simulink model "METI_Thermal_ver01_Jmaab_2018b"  (R2018b)
settings: Solver=ode8  StartTime=0  StopTime=end_time  FixedStep=sampling_time  RelTol=1e-3
PreLoadFcn:
  | %init_setting;
values from neighbouring files (symbols this model uses):
  degC2K = 273.15    [METI_TRAMI_Thermal_ver01_Jmaab_PreLoad.m]    (also in init_setting_METI.m)
  K2degC = -273.15    [METI_TRAMI_Thermal_ver01_Jmaab_PreLoad.m]    (also in init_setting_METI.m)
  sampling_time = 0.0025    [METI_TRAMI_Thermal_ver01_Jmaab_PreLoad.m]
undefined symbols (not defined in the file or in its folder): ACC_D_Gain, ACC_I_Gain, ACC_P_Gain, ALT_CNT_ALT_OFF_RPM_HYS_rpm, ALT_CNT_ALT_ON_RPM_HYS_rpm, ALT_CNT_Alter_V_BASE_V, ALT_CNT_Alter_V_Kaisei_V, ALT_CNT_flag_disable_kaisei, ALT_CNT_V_Battely_Kudo_V, ALT_PNT_ALT_GDCurrent_A, ALT_PNT_ALT_GDVolt_V, ALT_PNT_Alter_limit_Current_V_table, ALT_PNT_Alter_limit_Current_V_table_x_rpm, ALT_PNT_Alter_trq_Nm_map, ALT_PNT_Alter_trq_Nm_map_x_rpm, ALT_PNT_Alter_trq_Nm_map_y_Current_A, ALT_PNT_Alter_trq_Nm_map_z_Volt_tgt_V, ALT_PNT_eta_pulley_alt, ALT_PNT_Gain_Alt_v_del, ALT_PNT_ratio_pulley_alt, ALT_PNT_Tau_Alternator_V_tgt_s, ALT_PNT_trq_alter_output_LL_Nm, BK_PNT_Pow_UL, BK_PNT_Tau_brake, Brk_LL, Brk_PGain, Brk_UL, BT_PNT_Lo_Capa_lo_batt_F, BT_PNT_Lo_ocv_SOC_lo_batt_OCV_V_table, BT_PNT_Lo_ocv_SOC_lo_batt_OCV_V_table_x_SOC, BT_PNT_Lo_R_lo_batt_ohm, BT_PNT_Lo_SOC_MAX_lo_batt, BT_PNT_Lo_SOC_MIN_lo_batt, BT_PNT_Lo_SOC_START_lo_batt, BT_PNT_Lo_V_start_ocv, DF_PNT_DF_gear, DF_PNT_DFBlock2DFAir_Heat_Resi_KpW, DF_PNT_DFBlock_Heat_Capa_JpK, DF_PNT_DFBlock_Temp_ini_degC, DF_PNT_DFOil2DFBlock_Heat_Resi_KpW, DF_PNT_DFOil_Heat_Capa_JpK, DF_PNT_DFOil_Temp_ini_degC, DF_PNT_Driveshaft_damper, DF_PNT_Driveshaft_delta_radps_LL, DF_PNT_Driveshaft_delta_radps_UL, DF_PNT_Driveshaft_spring, DF_PNT_eta_DF, DF_PNT_Outtemp_degC, DF_PNT_TMBlock2DFBlock_Heat_Resi_KpW, Driver_Brake_Const1, Driver_Brake_Const3, Driver_Brake_Switch_Const2, Driver_Brk_sh, drivmode_ACC, drivmode_CONST, drivmode_GensokuKaisei, drivmode_GensokuRikko, drivmode_STOP, EL_PNT_R_bodyelec_lo_ohm, ENG_CNT_acc_idlestop ... (+137)
libraries: METI_Lib_vehicle_model x31, simulink x7, AZAPA_Lib_vehicle_model x1
(part 4 of 4)

== system METI_Thermal_ver01_Jmaab_2018b/Vehicle/CNT/ENG_CNT/ENG_Cntrl/Caliculate_Idle_Speed/Subsystem1 ==
  note: アイドル回転数時のFB
  omg_tgt_idle : Inport
  n_eng_rpm : Inport  Port=2
  per_throttle_base : Inport  Port=3
  flag_Lockup : Inport  Port=4
  flag_IdleStop : Inport  Port=5
  Logical Operator : Logic  Operator=OR  AllPortsSameDT=off  OutDataTypeStr=boolean
  Logical Operator1 : Logic  Operator=NOT  AllPortsSameDT=off  OutDataTypeStr=boolean
  Logical Operator2 : Logic  Inputs=3  AllPortsSameDT=off  OutDataTypeStr=boolean
  Logical Operator3 : Logic  Operator=NOT  AllPortsSameDT=off  OutDataTypeStr=boolean
  Logical Operator4 : Logic  Operator=NOT  AllPortsSameDT=off  OutDataTypeStr=boolean
  Logical Operator5 : Logic  AllPortsSameDT=off  OutDataTypeStr=boolean
  Relational Operator : RelationalOperator  Operator=<  OutDataTypeStr=boolean  RndMeth=Nearest
  Relational Operator2 : RelationalOperator  Operator=>  OutDataTypeStr=boolean  RndMeth=Nearest
  per_throttle_isc_fb : Constant  Value=ENG_CNT_per_throttle_isc_fb
  flag_idle_fb : Outport
  wires:
  per_throttle_base/1 -> Relational Operator/1
  per_throttle_isc_fb/1 -> Relational Operator/2
  Relational Operator2/1 -> Logical Operator2/1
  Relational Operator/1 -> Logical Operator1/1, Logical Operator5/1
  Logical Operator1/1 -> Logical Operator2/2
  Logical Operator5/1 -> Logical Operator/2
  flag_Lockup/1 -> Logical Operator3/1
  Logical Operator3/1 -> Logical Operator2/3
  Logical Operator2/1 -> Logical Operator/1
  omg_tgt_idle/1 -> Relational Operator2/1
  n_eng_rpm/1 -> Relational Operator2/2
  flag_IdleStop/1 -> Logical Operator4/1
  Logical Operator4/1 -> Logical Operator5/2
  Logical Operator/1 -> flag_idle_fb/1

== system METI_Thermal_ver01_Jmaab_2018b/Vehicle/PTTH/DTTH_PNT/DFTH_PNT/DFBlock_Heat_Capacity/degC->K ==
  degC : Inport
  Constant2 : Constant  Value=degC2K
  Sum : Sum  Inputs=++|
  K : Outport
  wires:
  degC/1 -> Sum/2
  Constant2/1 -> Sum/1
  Sum/1 -> K/1

== system METI_Thermal_ver01_Jmaab_2018b/Vehicle/PTTH/DTTH_PNT/DFTH_PNT/DFOil_Heat_Capacity/degC->K ==
  degC : Inport
  Constant2 : Constant  Value=degC2K
  Sum : Sum  Inputs=++|
  K : Outport
  wires:
  degC/1 -> Sum/2
  Constant2/1 -> Sum/1
  Sum/1 -> K/1

== system METI_Thermal_ver01_Jmaab_2018b/Vehicle/PTTH/DTTH_PNT/TMTH_PNT/CVTF_Heat_Capacity/degC->K ==
  degC : Inport
  Constant2 : Constant  Value=degC2K
  Sum : Sum  Inputs=++|
  K : Outport
  wires:
  degC/1 -> Sum/2
  Constant2/1 -> Sum/1
  Sum/1 -> K/1

== system METI_Thermal_ver01_Jmaab_2018b/Vehicle/PTTH/DTTH_PNT/TMTH_PNT/TMBlock_Heat_Capacity/degC->K ==
  degC : Inport
  Constant2 : Constant  Value=degC2K
  Sum : Sum  Inputs=++|
  K : Outport
  wires:
  degC/1 -> Sum/2
  Constant2/1 -> Sum/1
  Sum/1 -> K/1

== system METI_Thermal_ver01_Jmaab_2018b/Vehicle/PTTH/ENGTH_PNT/Subsystem/Coolant_Heat_Capacity/degC->K ==
  degC : Inport
  Constant2 : Constant  Value=degC2K
  Sum : Sum  Inputs=++|
  K : Outport
  wires:
  degC/1 -> Sum/2
  Constant2/1 -> Sum/1
  Sum/1 -> K/1

== system METI_Thermal_ver01_Jmaab_2018b/Vehicle/PTTH/ENGTH_PNT/Subsystem/ENGBlock_Heat_Capacity/degC->K ==
  degC : Inport
  Constant2 : Constant  Value=degC2K
  Sum : Sum  Inputs=++|
  K : Outport
  wires:
  degC/1 -> Sum/2
  Constant2/1 -> Sum/1
  Sum/1 -> K/1

== system METI_Thermal_ver01_Jmaab_2018b/Vehicle/PTTH/ENGTH_PNT/Subsystem/ENGOil_Heat_Capacity/degC->K ==
  degC : Inport
  Constant2 : Constant  Value=degC2K
  Sum : Sum  Inputs=++|
  K : Outport
  wires:
  degC/1 -> Sum/2
  Constant2/1 -> Sum/1
  Sum/1 -> K/1

== system METI_Thermal_ver01_Jmaab_2018b/Vehicle/PTTH/ENGTH_PNT/Subsystem/ENGOil_Heat_Capacity1/degC->K ==
  degC : Inport
  Constant2 : Constant  Value=degC2K
  Sum : Sum  Inputs=++|
  K : Outport
  wires:
  degC/1 -> Sum/2
  Constant2/1 -> Sum/1
  Sum/1 -> K/1

== system METI_Thermal_ver01_Jmaab_2018b/Vehicle/PTTH/RDTH_PNT/Subsystem/ENGBlock2Coolant_Heat_Resistance/K->degC ==
  K : Inport
  Constant2 : Constant  Value=K2degC
  Sum : Sum  Inputs=++|
  degC : Outport
  wires:
  K/1 -> Sum/2
  Constant2/1 -> Sum/1
  Sum/1 -> degC/1

== system METI_Thermal_ver01_Jmaab_2018b/Vehicle/PTTH/RDTH_PNT/Subsystem/RDCoolant_Heat_Capacity/degC->K ==
  degC : Inport
  Constant2 : Constant  Value=degC2K
  Sum : Sum  Inputs=++|
  K : Outport
  wires:
  degC/1 -> Sum/2
  Constant2/1 -> Sum/1
  Sum/1 -> K/1

== system METI_Thermal_ver01_Jmaab_2018b/Vehicle/TM_PNT/TM_PNT/TC_PNT/T_C/Cal_C_Capacity ==
  note: 容量係数
      | 加速中は＋
      | 減速中は－
  note: capacity coefficient
  note: N・m/rpm2
  ratio_n : Inport
  flag_acc_del : Inport  Port=2
  Product2 : Product  RndMeth=Zero
  ×10＾-6 : Gain  Gain=TM_PNT_ConvUnit
  容量係数 Lookup Table1 : Lookup_n-D  NumberOfTableDimensions=1  BreakpointsForDimension1=TM_PNT_torque_capacity_Nmprpm2_table_x_speed_ratio  Table=TM_PNT_torque_capacity_Nmprpm2_table  RndMeth=Simplest  InputSameDT=on
  c_capacity : Outport
  wires:
  容量係数 Lookup Table1/1 -> ×10＾-6/1
  ×10＾-6/1 -> Product2/1
  ratio_n/1 -> 容量係数 Lookup Table1/1
  Product2/1 -> c_capacity/1
  flag_acc_del/1 -> Product2/2

== system METI_Thermal_ver01_Jmaab_2018b/Vehicle/TM_PNT/TM_PNT/TC_PNT/T_C/Cal_Ratio_n ==
  n_TM_PNT_rpm : Inport
  n_GR_rpm : Inport  Port=2
  Compare To Constant1 : simulink/Logic and Bit Operations/Compare To Constant  relop=<=  const=TM_PNT_n_TC_min_rpm  OutDataTypeStr=boolean
  Compare To Constant2 : simulink/Logic and Bit Operations/Compare To Constant  relop=<=  const=TM_PNT_n_TC_min_rpm  OutDataTypeStr=boolean
  Constant : Constant  Value=0
  Logical Operator1 : Logic  Operator=OR  AllPortsSameDT=off  OutDataTypeStr=boolean
  MinMax : MinMax  Inputs=2
  Saturation1 : Saturate  UpperLimit=TM_PNT_w_ROT_T_C_UL  LowerLimit=TM_PNT_w_ROT_T_C_LL
  Saturation2 : Saturate  UpperLimit=TM_PNT_w_ROT_T_C_UL  LowerLimit=TM_PNT_w_ROT_T_C_LL
  Saturation5 : Saturate  UpperLimit=TM_PNT_ratio_w_ROT_T_C_UL  LowerLimit=TM_PNT_ratio_w_ROT_T_C_LL
  Subsystem : Subsystem
  Switch : Switch  Threshold=0.5
  加速時速度比 : Product  Inputs=*/
  減速時速度比 : Product  Inputs=*/
  ratio_n : Outport
  flag_acc_del : Outport  Port=2
  wires:
  Saturation2/1 -> 減速時速度比/1, 加速時速度比/2
  Saturation1/1 -> 減速時速度比/2, 加速時速度比/1
  加速時速度比/1 -> MinMax/1
  減速時速度比/1 -> MinMax/2
  MinMax/1 -> Saturation5/1
  Saturation5/1 -> Switch/3
  Constant/1 -> Switch/1
  Compare To Constant2/1 -> Logical Operator1/1
  Compare To Constant1/1 -> Logical Operator1/2
  Logical Operator1/1 -> Switch/2
  Switch/1 -> ratio_n/1
  n_GR_rpm/1 -> Subsystem/2(omg_tm), Saturation1/1, Compare To Constant1/1  "omg_tm"
  n_TM_PNT_rpm/1 -> Compare To Constant2/1, Subsystem/1(omg_engine), Saturation2/1  "omg_engine"
  Subsystem/1(flag_acc_del) -> flag_acc_del/1

== system METI_Thermal_ver01_Jmaab_2018b/Vehicle/TM_PNT/TM_PNT/TC_PNT/T_C/Cal_trq_TC_eng ==
  "n_TM_PNT_rpm " : Inport
  c_capacity : Inport  Port=2
  Math Function : Math  Operator=magnitude^2  SaturateOnIntegerOverflow=on
  Product : Product  RndMeth=Zero
  trq_TC_Nm : Outport
  wires:
  Product/1 -> trq_TC_Nm/1
  Math Function/1 -> Product/1
  c_capacity/1 -> Product/2
  "n_TM_PNT_rpm "/1 -> Math Function/1

== system METI_Thermal_ver01_Jmaab_2018b/Vehicle/TM_PNT/TM_PNT/TC_PNT/T_C/Cal_Ratio_n/Subsystem ==
  note: エンジン加速中は1、減速中は-1
  omg_engine : Inport
  omg_tm : Inport  Port=2
  Saturation : Saturate  UpperLimit=1  LowerLimit=-1
  Subtract : Sum  Inputs=-+|
  flag_acc_del : Outport
  wires:
  Subtract/1 -> Saturation/1
  Saturation/1 -> flag_acc_del/1
  omg_tm/1 -> Subtract/1
  omg_engine/1 -> Subtract/2
